simulink model "Three_Phase_DiodeRectifier_Rload"  (R2018b)
settings: Solver=VariableStepAuto  StartTime=0.0  StopTime=0.1  RelTol=1e-3
libraries: powerlib x19
settings Model: Creator=A.hey  LastModifiedBy=A.hey

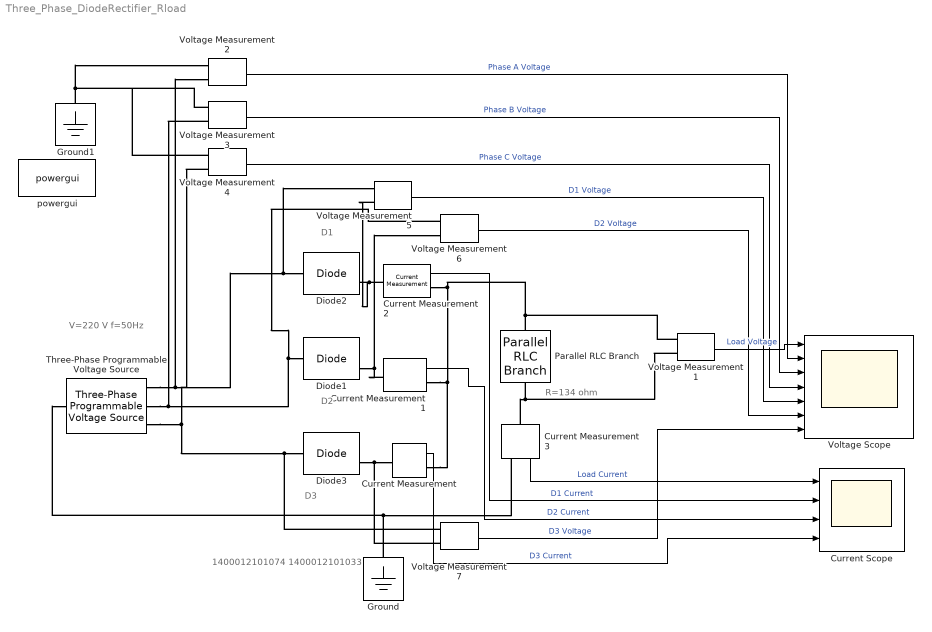
== system Three_Phase_DiodeRectifier_Rload ==
  note: V=220 V
      | f=50Hz
  note: 1400012101074
      | 1400012101033
  note: R=134 ohm
  note: D1
  note: D2
  note: D3
  Current Measurement{,1..3} (4 alike) : powerlib/Measurements/Current Measurement  PhasorSimulation=off  OutputType=Complex  PSBequivalent=0
  Current Scope : Scope  NumInputPorts=4
  Diode1 : powerlib/Power Electronics/Diode  Ron=0.001  Lon=0  Vf=0.8  IC=0  UseSnubber=0  Rs=500  Cs=250e-9  Measurements=on
  Diode2 : powerlib/Power Electronics/Diode  Ron=0.001  Lon=0  Vf=0.8  IC=0  UseSnubber=0  Rs=500  Cs=250e-9  Measurements=on
  Diode3 : powerlib/Power Electronics/Diode  Ron=0.001  Lon=0  Vf=0.8  IC=0  UseSnubber=0  Rs=500  Cs=250e-9  Measurements=on
  Ground : powerlib/Elements/Ground  LConnTagsString=a
  Ground1 : powerlib/Elements/Ground  LConnTagsString=a
  Parallel RLC Branch : powerlib/Elements/Parallel RLC Branch  LConnTagsString=a  RConnTagsString=__new0  BranchType=R  Resistance=134  Inductance=1e-3  SetiL0=off  InitialCurrent=0  Capacitance=1e-6  Setx0=off  InitialVoltage=0  Measurements=None
  Three-Phase Programmable Voltage Source : powerlib/Electrical Sources/Three-Phase Programmable Voltage Source  PositiveSequence="[220  0 50]"  VariationEntity=None  VariationType=Table of time-amplitude pairs  VariationTypeAlt=Step  VariationStep=0.5  VariationRate=10  VariationMagnitude=0.3  VariationFrequency=2  VariationTiming=[1 2]  VariationPhaseA=off  Amplitudes=[1 0.8 1.2 1.0]  TimeValues=[0 0.1 0.15 0.2]  HarmonicGeneration=off  HarmonicA=[3 0.2 -25 0]  HarmonicB=[2 0.15 35 2]  Timing="[0.05  3]"  BusType=swing  Pref=0  Qref=0  Qmin=-inf  Qmax=inf
  Voltage Measurement{1..7} (7 alike) : powerlib/Measurements/Voltage Measurement  PhasorSimulation=off  OutputType=Complex  PSBequivalent=0
  "Voltage Scope " : Scope  NumInputPorts=7
  powergui : powerlib/powergui  Priority=1  SimulationMode=Continuous  SampleTime=50e-6  frequency=60  Iterations=50  frequencyindice=50  Pbase=100e6  ErrMax=1e-4  UnitsV=kV  UnitsW=MW  buscounter=0  FunctionMessages=off  echomessages=off  EnableUseOfTLC=off  CurrentSourceSwitches=off  DisableSnubberDevices=off  DisableRonSwitches=off  DisableVfSwitches=off  DisplayEquations=off  SolverType=Tustin/Backward Euler (TBE)  Interpol=off  ExternalGateDelay=off  methode=off  Ts=100  x0status=blocks  SPID=on  SwTol=0  HookPort=off  RestoreLinks=warning  ResistiveCurrentMeasurement=off  Frange=[0:2:500]  Ylog=off  Xlog=on  ShowGrid=off  save=off  variable=ZData  structure=0  ZoomFFT=off  StartTime=0.0  cycles=1  DisplayStyle=1  fundamental=60  FreqAxis=off  MaxFrequency=1000  frequencyindicesteady=1  RmsSteady=1  display=off
  wires:
  Voltage Measurement1/1 -> "Voltage Scope "/1  "Load Voltage"
  Voltage Measurement2/1 -> "Voltage Scope "/2  "Phase A Voltage"
  Voltage Measurement3/1 -> "Voltage Scope "/3  "Phase B Voltage"
  Voltage Measurement4/1 -> "Voltage Scope "/4  "Phase C Voltage"
  Voltage Measurement5/1 -> "Voltage Scope "/5  "D1 Voltage"
  Voltage Measurement6/1 -> "Voltage Scope "/6  "D2 Voltage"
  Voltage Measurement7/1 -> "Voltage Scope "/7  "D3 Voltage"
  Current Measurement3/1 -> Current Scope/1  "Load Current"
  Current Measurement2/1 -> Current Scope/2  "D1 Current"
  Current Measurement1/1 -> Current Scope/3  "D2 Current"
  Current Measurement/1 -> Current Scope/4  "D3 Current"
  connections:
  Three-Phase Programmable Voltage Source/RConn3 -- Voltage Measurement4/LConn1 -- Voltage Measurement7/LConn1 -- Diode3/LConn1
  Three-Phase Programmable Voltage Source/RConn2 -- Voltage Measurement3/LConn1 -- Voltage Measurement6/LConn1 -- Diode1/LConn1
  Three-Phase Programmable Voltage Source/RConn1 -- Diode2/LConn1 -- Voltage Measurement5/LConn1 -- Voltage Measurement2/LConn1
  Parallel RLC Branch/LConn1 -- Current Measurement/RConn1 -- Current Measurement1/RConn1 -- Current Measurement2/RConn1 -- Voltage Measurement1/LConn1
  Voltage Measurement1/LConn2 -- Current Measurement3/LConn1 -- Parallel RLC Branch/RConn1
  Diode3/RConn1 -- Voltage Measurement7/LConn2 -- Current Measurement/LConn1
  Current Measurement1/LConn1 -- Voltage Measurement6/LConn2 -- Diode1/RConn1
  Current Measurement2/LConn1 -- Diode2/RConn1 -- Voltage Measurement5/LConn2
  Ground/LConn1 -- Three-Phase Programmable Voltage Source/LConn1 -- Current Measurement3/RConn1
  Ground1/LConn1 -- Voltage Measurement4/LConn2 -- Voltage Measurement3/LConn2 -- Voltage Measurement2/LConn2
